simulink model "ivedsp2"  (Simulink 7.6)
settings: Solver=FixedStepDiscrete  StartTime=0.0  StopTime=10  FixedStep=1  RelTol=1e-3
libraries: simulink x17
settings Model: Creator=jordan  LastModifiedBy=jordan
settings DataIOCC: LimitDataPoints=off  SaveOutput=off  SignalLogging=off  DSMLogging=off  SaveTime=off
settings OptimizationCC: BlockReduction=off  ConditionallyExecuteInputs=off  InlineParams=on

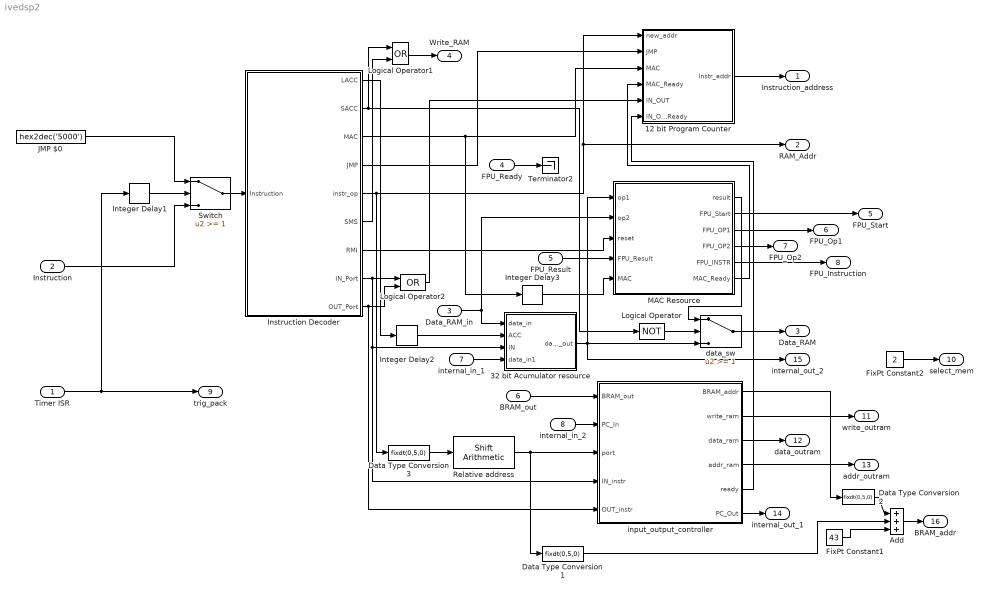
== system ivedsp2 ==
  Timer ISR : Inport  OutDataTypeStr=boolean
  Instruction : Inport  Port=2  OutDataTypeStr=uint16
  Data_RAM_in : Inport  Port=3  OutDataTypeStr=uint32
  FPU_Ready : Inport  Port=4  OutDataTypeStr=boolean
  FPU_Result : Inport  Port=5  OutDataTypeStr=uint32
  BRAM_out : Inport  Port=6  OutDataTypeStr=uint8
  internal_in_1 : Inport  Port=7  OutDataTypeStr=uint32
  internal_in_2 : Inport  Port=8  OutDataTypeStr=uint8  PortDimensions=4
  12 bit Program Counter : Subsystem
  32 bit Acumulator resource : Subsystem
  Add : Sum  Inputs=+++  AccumDataTypeStr=fixdt(0,11,0)  OutDataTypeStr=fixdt(0,11,0)
  Data Type Conversion1 : DataTypeConversion  OutDataTypeStr=fixdt(0,5,0)
  Data Type Conversion2 : DataTypeConversion  OutDataTypeStr=fixdt(0,5,0)
  Data Type Conversion3 : DataTypeConversion  OutDataTypeStr=fixdt(0,5,0)
  FixPt Constant1 : Constant  DisableCoverage=on  Value=43  OutDataTypeStr=fixdt(0,11,0)
  FixPt Constant2 : Constant  DisableCoverage=on  Value=2  OutDataTypeStr=fixdt(0,4,0)
  Instruction Decoder : Subsystem
  Integer Delay1 : simulink/Discrete/Integer Delay  NumDelays=1  vinit=0.0  samptime=-1
  Integer Delay2 : simulink/Discrete/Integer Delay  NumDelays=1  vinit=0.0  samptime=-1
  Integer Delay3 : simulink/Discrete/Integer Delay  NumDelays=1  vinit=0.0  samptime=-1
  JMP $0 : Constant  DisableCoverage=on  Value=hex2dec('5000')  OutDataTypeStr=Inherit: Inherit via back propagation
  Logical Operator : Logic  Operator=NOT  AllPortsSameDT=off  OutDataTypeStr=boolean
  Logical Operator1 : Logic  Operator=OR  AllPortsSameDT=off  OutDataTypeStr=boolean
  Logical Operator2 : Logic  Operator=OR  AllPortsSameDT=off  OutDataTypeStr=boolean
  MAC Resource : Stateflow chart  TreatAsAtomicUnit=on
  Relative address : simulink/Logic and Bit Operations/Shift Arithmetic  SystemSampleTime=-1  nBitShiftRight=-2  nBinPtShiftRight=0
  Switch : Switch  Threshold=1
  Terminator2 : Terminator
  data_sw : Switch  Threshold=1
  input_output_controller : Stateflow chart  TreatAsAtomicUnit=on
  Instruction_address : Outport  OutDataTypeStr=fixdt(0,12,0)
  RAM_Addr : Outport  Port=2  OutDataTypeStr=fixdt(0,12,0)
  Data_RAM : Outport  Port=3  OutDataTypeStr=uint32
  Write_RAM : Outport  Port=4  OutDataTypeStr=boolean
  FPU_Start : Outport  Port=5  OutDataTypeStr=boolean
  FPU_Op1 : Outport  Port=6  OutDataTypeStr=uint32
  FPU_Op2 : Outport  Port=7  OutDataTypeStr=uint32
  FPU_Instruction : Outport  Port=8  OutDataTypeStr=fixdt(0,3,0)
  trig_pack : Outport  Port=9
  select_mem : Outport  Port=10
  write_outram : Outport  Port=11
  data_outram : Outport  Port=12
  addr_outram : Outport  Port=13
  internal_out_1 : Outport  Port=14
  internal_out_2 : Outport  Port=15  OutDataTypeStr=uint32
  BRAM_addr : Outport  Port=16
  wires:
  MAC Resource/1(result) -> data_sw/1
  32 bit Acumulator resource/1(data_out) -> data_sw/3, MAC Resource/1(op1), internal_out_2/1
  Data_RAM_in/1 -> 32 bit Acumulator resource/1(data_in), MAC Resource/2(op2)
  Instruction Decoder/5(instr_op) -> 12 bit Program Counter/1(new_addr), RAM_Addr/1, Data Type Conversion3/1
  Instruction Decoder/1(LACC) -> Integer Delay2/1
  Integer Delay2/1 -> 32 bit Acumulator resource/2(ACC)
  Instruction Decoder/2(SACC) -> Logical Operator/1, Logical Operator1/1
  Logical Operator/1 -> data_sw/2
  Instruction Decoder/4(JMP) -> 12 bit Program Counter/2(JMP)
  Instruction Decoder/3(MAC) -> 12 bit Program Counter/3(MAC), Integer Delay3/1
  Instruction Decoder/7(RMI) -> MAC Resource/3(reset)
  Instruction Decoder/6(SMS) -> Logical Operator1/2
  Instruction Decoder/8(IN_Port) -> input_output_controller/4(IN_instr), 32 bit Acumulator resource/3(IN), Logical Operator2/1
  Data Type Conversion3/1 -> Relative address/1
  Switch/1 -> Instruction Decoder/1(Instruction)
  JMP $0/1 -> Switch/1
  12 bit Program Counter/1(Instr_addr) -> Instruction_address/1
  Instruction/1 -> Switch/3
  data_sw/1 -> Data_RAM/1
  Logical Operator1/1 -> Write_RAM/1
  FPU_Result/1 -> MAC Resource/4(FPU_Result)
  MAC Resource/3(FPU_OP1) -> FPU_Op1/1
  MAC Resource/4(FPU_OP2) -> FPU_Op2/1
  MAC Resource/5(FPU_INSTR) -> FPU_Instruction/1
  MAC Resource/2(FPU_Start) -> FPU_Start/1
  Instruction Decoder/9(OUT_Port) -> Logical Operator2/2, input_output_controller/5(OUT_instr)
  BRAM_out/1 -> input_output_controller/1(BRAM_out)
  input_output_controller/4(addr_ram) -> addr_outram/1
  input_output_controller/2(write_ram) -> write_outram/1
  input_output_controller/3(data_ram) -> data_outram/1
  input_output_controller/1(BRAM_addr) -> Data Type Conversion2/1
  Relative address/1 -> input_output_controller/3(port), Data Type Conversion1/1
  input_output_controller/5(ready) -> 12 bit Program Counter/6(IN_OUT_Ready)
  MAC Resource/6(MAC_Ready) -> 12 bit Program Counter/4(MAC_Ready)
  Logical Operator2/1 -> 12 bit Program Counter/5(IN_OUT)
  internal_in_1/1 -> 32 bit Acumulator resource/4(data_in1)
  internal_in_2/1 -> input_output_controller/2(PC_In)
  Integer Delay1/1 -> Switch/2
  FPU_Ready/1 -> Terminator2/1
  input_output_controller/6(PC_Out) -> internal_out_1/1
  Add/1 -> BRAM_addr/1
  Data Type Conversion1/1 -> Add/2
  FixPt Constant1/1 -> Add/3
  FixPt Constant2/1 -> select_mem/1
  Timer ISR/1 -> trig_pack/1, Integer Delay1/1
  Data Type Conversion2/1 -> Add/1
  Integer Delay3/1 -> MAC Resource/5(MAC)

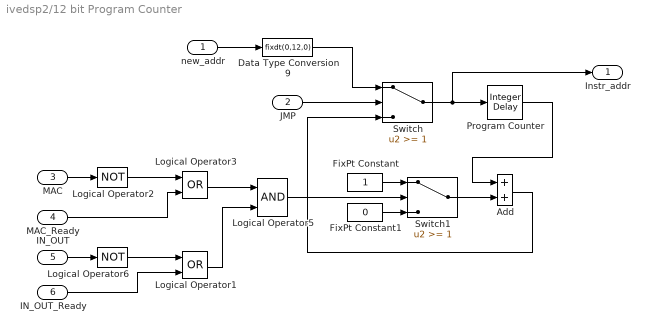
== system ivedsp2/12 bit Program Counter ==
  new_addr : Inport
  JMP : Inport  Port=2
  MAC : Inport  Port=3  OutDataTypeStr=boolean
  MAC_Ready : Inport  Port=4  OutDataTypeStr=boolean
  IN_OUT : Inport  Port=5  OutDataTypeStr=boolean
  IN_OUT_Ready : Inport  Port=6  OutDataTypeStr=boolean
  Add : Sum  AccumDataTypeStr=fixdt(0,12,0)  OutDataTypeStr=fixdt(0,12,0)
  Data Type Conversion9 : DataTypeConversion  OutDataTypeStr=fixdt(0,12,0)
  FixPt Constant : Constant  DisableCoverage=on  OutDataTypeStr=fixdt(0,12,0)
  FixPt Constant1 : Constant  DisableCoverage=on  Value=0  OutDataTypeStr=fixdt(0,12,0)
  Logical Operator1 : Logic  Operator=OR  AllPortsSameDT=off  OutDataTypeStr=boolean
  Logical Operator2 : Logic  Operator=NOT  AllPortsSameDT=off  OutDataTypeStr=boolean
  Logical Operator3 : Logic  Operator=OR  AllPortsSameDT=off  OutDataTypeStr=boolean
  Logical Operator5 : Logic  AllPortsSameDT=off  OutDataTypeStr=boolean
  Logical Operator6 : Logic  Operator=NOT  AllPortsSameDT=off  OutDataTypeStr=boolean
  Program Counter : simulink/Discrete/Integer Delay  NumDelays=1  vinit=0.0  samptime=-1
  Switch : Switch  Threshold=1
  Switch1 : Switch  Threshold=1
  Instr_addr : Outport  InitialOutput=0
  wires:
  JMP/1 -> Switch/2
  new_addr/1 -> Data Type Conversion9/1
  Program Counter/1 -> Add/1
  Switch/1 -> Program Counter/1, Instr_addr/1
  FixPt Constant/1 -> Switch1/1
  Add/1 -> Switch/3
  Data Type Conversion9/1 -> Switch/1
  Switch1/1 -> Add/2
  FixPt Constant1/1 -> Switch1/3
  Logical Operator3/1 -> Logical Operator5/1
  Logical Operator2/1 -> Logical Operator3/1
  MAC/1 -> Logical Operator2/1
  MAC_Ready/1 -> Logical Operator3/2
  Logical Operator1/1 -> Logical Operator5/2
  Logical Operator6/1 -> Logical Operator1/1
  IN_OUT/1 -> Logical Operator6/1
  IN_OUT_Ready/1 -> Logical Operator1/2
  Logical Operator5/1 -> Switch1/2

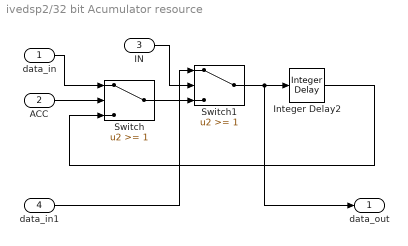
== system ivedsp2/32 bit Acumulator resource ==
  data_in : Inport
  ACC : Inport  Port=2
  IN : Inport  Port=3
  data_in1 : Inport  Port=4
  Integer Delay2 : simulink/Discrete/Integer Delay  NumDelays=1  vinit=0.0  samptime=-1
  Switch : Switch  Threshold=1
  Switch1 : Switch  Threshold=1
  data_out : Outport  OutDataTypeStr=uint32
  wires:
  Switch/1 -> Switch1/3
  Integer Delay2/1 -> Switch/3
  data_in/1 -> Switch/1
  ACC/1 -> Switch/2
  Switch1/1 -> Integer Delay2/1, data_out/1
  IN/1 -> Switch1/2
  data_in1/1 -> Switch1/1

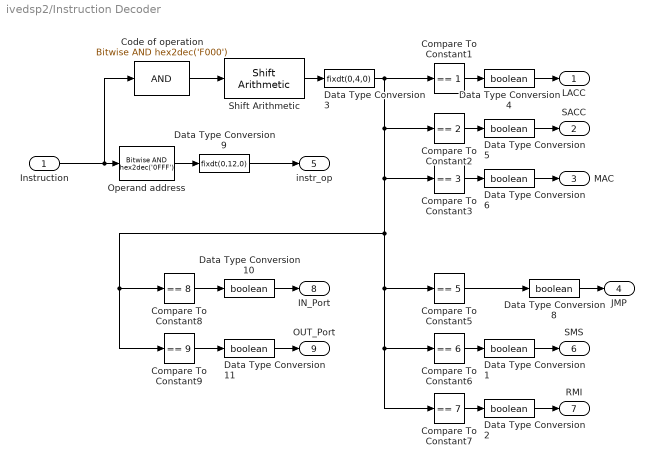
== system ivedsp2/Instruction Decoder ==
  Instruction : Inport  OutDataTypeStr=uint16
  Code of operation : simulink/Logic and Bit Operations/Bitwise Operator  logicop=AND  UseBitMask=on  BitMask=hex2dec('F000')  BitMaskRealWorld=Stored Integer
  Compare To Constant1 : simulink/Logic and Bit Operations/Compare To Constant  SystemSampleTime=-1  relop===  const=1  LogicOutDataTypeMode=boolean
  Compare To Constant2 : simulink/Logic and Bit Operations/Compare To Constant  SystemSampleTime=-1  relop===  const=2  LogicOutDataTypeMode=boolean
  Compare To Constant3 : simulink/Logic and Bit Operations/Compare To Constant  SystemSampleTime=-1  relop===  const=3  LogicOutDataTypeMode=boolean
  Compare To Constant5 : simulink/Logic and Bit Operations/Compare To Constant  SystemSampleTime=-1  relop===  const=5  LogicOutDataTypeMode=boolean
  Compare To Constant6 : simulink/Logic and Bit Operations/Compare To Constant  SystemSampleTime=-1  relop===  const=6  LogicOutDataTypeMode=boolean
  Compare To Constant7 : simulink/Logic and Bit Operations/Compare To Constant  SystemSampleTime=-1  relop===  const=7  LogicOutDataTypeMode=boolean
  Compare To Constant8 : simulink/Logic and Bit Operations/Compare To Constant  SystemSampleTime=-1  relop===  const=8  LogicOutDataTypeMode=boolean
  Compare To Constant9 : simulink/Logic and Bit Operations/Compare To Constant  SystemSampleTime=-1  relop===  const=9  LogicOutDataTypeMode=boolean
  Data Type Conversion{1..2,4..6,8,10..11} (8 alike) : DataTypeConversion  OutDataTypeStr=boolean
  Data Type Conversion3 : DataTypeConversion  OutDataTypeStr=fixdt(0,4,0)
  Data Type Conversion9 : DataTypeConversion  OutDataTypeStr=fixdt(0,12,0)
  Operand address : simulink/Logic and Bit Operations/Bitwise Operator  logicop=AND  UseBitMask=on  BitMask=hex2dec('0FFF')  BitMaskRealWorld=Stored Integer
  Shift Arithmetic : simulink/Logic and Bit Operations/Shift Arithmetic  SystemSampleTime=-1  nBitShiftRight=12  nBinPtShiftRight=0
  LACC : Outport
  SACC : Outport  Port=2
  MAC : Outport  Port=3
  JMP : Outport  Port=4
  instr_op : Outport  Port=5
  SMS : Outport  Port=6
  RMI : Outport  Port=7
  IN_Port : Outport  Port=8
  OUT_Port : Outport  Port=9
  wires:
  Instruction/1 -> Operand address/1, Code of operation/1
  Code of operation/1 -> Shift Arithmetic/1
  Shift Arithmetic/1 -> Data Type Conversion3/1
  Data Type Conversion3/1 -> Compare To Constant6/1, Compare To Constant7/1, Compare To Constant5/1, Compare To Constant8/1, Compare To Constant9/1, Compare To Constant3/1, Compare To Constant2/1, Compare To Constant1/1
  Compare To Constant1/1 -> Data Type Conversion4/1
  Compare To Constant2/1 -> Data Type Conversion5/1
  Compare To Constant3/1 -> Data Type Conversion6/1
  Compare To Constant5/1 -> Data Type Conversion8/1
  Operand address/1 -> Data Type Conversion9/1
  Data Type Conversion4/1 -> LACC/1
  Data Type Conversion5/1 -> SACC/1
  Data Type Conversion9/1 -> instr_op/1
  Data Type Conversion6/1 -> MAC/1
  Data Type Conversion8/1 -> JMP/1
  Compare To Constant6/1 -> Data Type Conversion1/1
  Data Type Conversion1/1 -> SMS/1
  Compare To Constant7/1 -> Data Type Conversion2/1
  Data Type Conversion2/1 -> RMI/1
  Compare To Constant8/1 -> Data Type Conversion10/1
  Data Type Conversion10/1 -> IN_Port/1
  Compare To Constant9/1 -> Data Type Conversion11/1
  Data Type Conversion11/1 -> OUT_Port/1

== stateflow chart MAC Resource ==
  settings: executeAtInitialization=1
  state Multipy
  state Multipy2
  state Wait
  state Wait3
  state Accumulate1
  state Accumulate2
  state Multipy1
  state Accumulate3
  state Multipy3
  (default) -> Wait : {result=0;}
  Multipy3 -> Multipy : {FPU_OP1=buf_op1;
      | FPU_OP2=buf_op2;
      | FPU_INSTR=2;
      | FPU_Start=1;}
  (junction 13) -> Accumulate3 [order 1] : [ind==11]
      | {buf_res=FPU_Result;
      | ind=0;}
  (junction 14) -> Accumulate1 [order 2] : {ind++;}
  (junction 14) -> Multipy1 [order 1] : [ind==7]{
      | Internal_ACC=FPU_Result;}
  Wait -> (junction 12)
  (junction 12) -> Wait [order 1] : [reset]{
      | Internal_ACC=0;
      | result=0;
      | FPU_OP1=0;
      | FPU_OP2=0;}
  (junction 12) -> Wait [order 3]
  Accumulate2 -> Accumulate1 : {FPU_Start=0;
      | ind=0;}
  Multipy -> Wait3 : {FPU_Start=0;
      | ind=0;}
  Wait3 -> (junction 13)
  (junction 13) -> Wait3 [order 2] : {ind++;}
  Accumulate1 -> (junction 14)
  Accumulate3 -> Accumulate2 : {FPU_OP1=buf_res;
      | FPU_OP2=Internal_ACC;
      | FPU_INSTR=0;
      | FPU_Start=1;}
  Multipy1 -> Multipy2 : {result=Internal_ACC;
      | MAC_Ready=1;}
  Multipy2 -> Wait : {MAC_Ready=0;
      | FPU_OP1=0;
      | FPU_OP2=0;}
  (junction 12) -> Multipy3 [order 2] : [MAC]{
      | buf_op1=op1;
      | buf_op2=op2;}
  data: op1 input uint32; op2 input uint32; reset input boolean; Internal_ACC local uint32; result output uint32 =0; FPU_Start output boolean =0; FPU_OP1 output uint32 =0; FPU_OP2 output uint32 =0; FPU_Result input uint32; FPU_INSTR output fixdt(0,3,0) =0; MAC_Ready output boolean =0; ind local fixdt(0,4,0); buf_res local uint32; MAC input boolean; buf_op1 local uint32; buf_op2 local uint32

== stateflow chart input_output_controller ==
  settings: executeAtInitialization=1
  state IN_Wait
  state Receive
  state OUT_Wait
  state IN_Wait2
  state IN_Wait3
  state Wait
  state Wait4
  state Wait5
  state IN_Wait4
  state IN_Wait1
  state IN_Wait5
  state IN_Wait6
  state IN_Wait7
  state IN_Wait8
  IN_Wait5 -> IN_Wait : {PC_Outb[0]=BRAM_out;
      | BRAM_addr=1;}
  IN_Wait8 -> Wait4 : {PC_Outb[3]=BRAM_out;
      | ready=1;}
  Wait4 -> Wait5 : {ready=0;
      | PC_Out=PC_Outb;}
  (junction 64) -> Wait4 [order 1] : [ind==4]{
      | write_ram=0;
      | ready=1;}
  IN_Wait7 -> IN_Wait4 : {PC_Outb[2]=BRAM_out;
      | BRAM_addr=3;}
  Receive -> Wait [order 1] : [OUT_instr==1]{ready=0;}
  IN_Wait6 -> IN_Wait3 : {PC_Outb[1]=BRAM_out;
      | BRAM_addr=2;}
  (junction 64) -> OUT_Wait [order 2] : {addr_ram=addr_ram+1;
      | data_ram=PC_In[ind];}
  OUT_Wait -> (junction 64) : {ind++;}
  Wait5 -> Receive
  IN_Wait2 -> IN_Wait1 : {BRAM_addr=0;}
  Wait -> OUT_Wait : {addr_ram=port;
      | write_ram=1;
      | data_ram=PC_In[0];
      | ind=0;}
  (default) -> Receive
  Receive -> IN_Wait2 [order 2] : [IN_instr==1]{ready=0;}
  IN_Wait1 -> IN_Wait5
  IN_Wait -> IN_Wait6
  IN_Wait3 -> IN_Wait7
  IN_Wait4 -> IN_Wait8
  data: BRAM_out input uint8; BRAM_addr output fixdt(0,2,0) =0; ind local fixdt(0,5,0) =0; LastCmd local uint8; packet_out local uint8 size=16; write_ram output boolean =0; data_ram output uint8; addr_ram output fixdt(0,14,0) =0; PC_In input uint8 size=4; PC_Outb local uint8 size=4; port input fixdt(0,5,0); IN_instr input boolean; ready output boolean; OUT_instr input boolean; PC_Out output uint8 size=4
